simulink subsystem "kemba_simulation"  (R2022a)
settings: Solver=VariableStepAuto  StartTime=0.0  StopTime=10.0  RelTol=1e-3
values from neighbouring files (symbols this model uses):
  N = 6    [parameters.m]
undefined symbols (not defined in the file or in its folder): Body, Carrier, Femur, Piston, Ring, Tibia, X, Y, Z
libraries: sm_lib x95, nesl_utility x33, eeGeneralControl x4, Multibody_Parts_Lib x2, fl_lib x2
(part 4 of 4)

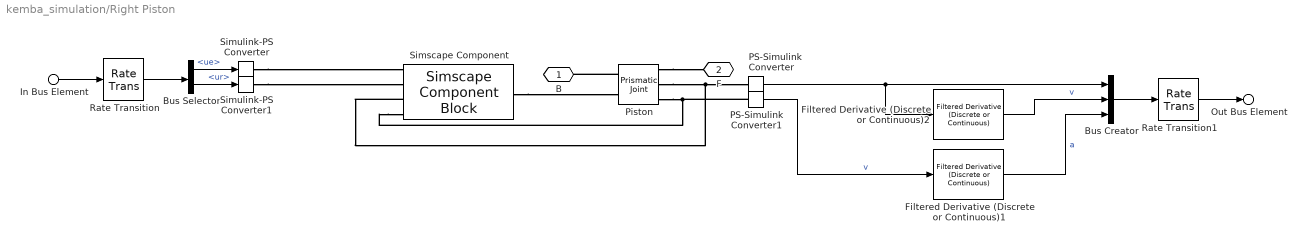
== system kemba_simulation/Right Piston ==
  In Bus Element : Inport  PortName=cmd
  Bus Creator : BusCreator  Inputs=3  OutDataTypeStr=Bus: PistonState
      settings: InheritFromInputs=off
  Bus Selector : BusSelector  OutputSignals=ue,ur
  Filtered Derivative (Discrete or Continuous)1 : eeGeneralControl/Filtered Derivative (Discrete or Continuous)  K=1  T=0.002  B=inf  A=-inf  minRatio=2  init_option=Inherited from block input  x0=0  Ts=-1
      settings: SourceProductBaseCode=PS
  Filtered Derivative (Discrete or Continuous)2 : eeGeneralControl/Filtered Derivative (Discrete or Continuous)  K=1  T=0.002  B=inf  A=-inf  minRatio=2  init_option=Inherited from block input  x0=0  Ts=-1
      settings: SourceProductBaseCode=PS
  PS-Simulink Converter : nesl_utility/PS-Simulink Converter  PhysicalDomain=network_engine_domain  SubClassName=ps_output  LeftPortType=input  RightPortType=output  PseudoPeriodic=off  Frequencies=[]  VectorFormat=inherit  Unit=inherit  AffineConversion=off
      settings: SourceProductBaseCode=SS,PW,VE
  PS-Simulink Converter1 : nesl_utility/PS-Simulink Converter  PhysicalDomain=network_engine_domain  SubClassName=ps_output  LeftPortType=input  RightPortType=output  PseudoPeriodic=off  Frequencies=[]  VectorFormat=inherit  Unit=inherit  AffineConversion=off
      settings: SourceProductBaseCode=SS,PW,VE
  Piston : sm_lib/Joints/Prismatic Joint  JointMode=Normal  SenseConstraintForce=off  SenseConstraintForceX=off  SenseConstraintForceY=off  SenseConstraintForceZ=off  SenseConstraintTorque=off  SenseConstraintTorqueX=off  SenseConstraintTorqueY=off  SenseConstraintTorqueZ=off  SenseTotalForce=off  SenseTotalForceX=off  SenseTotalForceY=off  SenseTotalForceZ=off  SenseTotalTorque=off  SenseTotalTorqueX=off  SenseTotalTorqueY=off  SenseTotalTorqueZ=off  CompositeWrenchDir=FollowerOnBase  CompositeWrenchFrame=BaseFrame  EquilibriumPosition=0  EquilibriumPositionUnits=m  SpringStiffness=0  SpringStiffnessUnits=N/m  DampingCoefficient=0  DampingCoefficientUnits=N/(m/s)  TorqueActuationMode=InputTorque  MotionActuationMode=ComputedMotion  SensePosition=on  SenseVelocity=on  SenseAcceleration=off  SenseTorqueForce=off  SenseLowerLimitTorqueForce=off  SenseUpperLimitTorqueForce=off  LowerLimitSpecify=on  LowerLimitBound=0  LowerLimitBoundUnits=m  LowerLimitStiffness=Piston.Limit.stiffness  LowerLimitStiffnessUnits=N/m  LowerLimitDamping=Piston.Limit.damping  LowerLimitDampingUnits=N/(m/s)  LowerLimitTransitionRegionWidth=Piston.Limit.transition_region_width  LowerLimitTransitionRegionWidthUnits=m  UpperLimitSpecify=on  UpperLimitBound=70  UpperLimitBoundUnits=mm  UpperLimitStiffness=Piston.Limit.stiffness  UpperLimitStiffnessUnits=N/m  UpperLimitDamping=Piston.Limit.damping  UpperLimitDampingUnits=N/(m/s)  UpperLimitTransitionRegionWidth=Piston.Limit.transition_region_width  UpperLimitTransitionRegionWidthUnits=m  PositionTargetSpecify=on  PositionTargetPriority=High  PositionTargetValue=Piston.Right.p0  PositionTargetValueUnits=m  VelocityTargetSpecify=on  VelocityTargetPriority=High  VelocityTargetValue=Piston.Right.v0  VelocityTargetValueUnits=m/s
  Rate Transition : RateTransition
  Rate Transition1 : RateTransition
  Simscape Component : SimscapeComponentBlock  SourceFile=PistonDynamics  ComponentPath=PistonDynamics  ComponentVariants="[\"PistonDynamics\"]"  ComponentVariantNames="[\"PistonDynamics\"]"  ClassName=PistonDynamics  SchemaVersion=1  Ps=7 bar  Pe=1 atm  Db=25 mm  Dr=10 mm  do=3 mm  td=6 ms  l=70 mm  kd=5 N  kv=25 N*s/m  T=295 K  R=286.71 J/(K*kg)  c=0.5  Z=0.99  k=1.4  v1=13069 mm^3  v2=16084 mm^3  P1_specify=off  P1_priority=None  P1=1 atm  P1_nominal_specify=off  P1_nominal_unit=atm  P1_nominal_value=1  P2_specify=off  P2_priority=None  P2=1 atm  P2_nominal_specify=off  P2_nominal_unit=atm  P2_nominal_value=1
      settings: CopyFcn=simscape.engine.sli.internal.componentblockcallback(gcbh,'COPY')  PreCopyFcn=simscape.engine.sli.internal.componentblockcallback(gcbh,'PRECOPY')  PreDeleteFcn=simscape.engine.sli.internal.componentblockcallback(gcbh,'PREDELETE')  LogSimulationData=on  InternalSimscapePortConfiguration="{\"Bottom\":[],\"Left\":[{\"id\":\"ue\",\"label\":\"ue\",\"type\":\"input\"},{\"id\":\"ur\",\"label\":\"ur\",\"type\":\"input\"},{\"id\":\"x\",\"label\":\"x\",\"type\":\"input\"},{\"id\":\"v\",\"label\":\"v\",\"type\":\"input\"}],\"Right\":[{\"id\":\"F\",\"label\":\"F\",\"type\":\"output\"}],\"Top\":[]}"
      mask Type: Piston Pressure Dynamics
  Simulink-PS Converter : nesl_utility/Simulink-PS Converter  PhysicalDomain=network_engine_domain  SubClassName=ps_input  LeftPortType=input  RightPortType=output  PseudoPeriodic=off  Frequencies=[]  NoiseDistribution=none  NoiseParameters=[]  Unit=1  AffineConversion=off  FilteringAndDerivatives=provide  SimscapeFilterOrder=1  InputFilterTimeConstant=0.001  UdotUserProvided=0
      settings: SourceProductBaseCode=SS,PW,VE
  Simulink-PS Converter1 : nesl_utility/Simulink-PS Converter  PhysicalDomain=network_engine_domain  SubClassName=ps_input  LeftPortType=input  RightPortType=output  PseudoPeriodic=off  Frequencies=[]  NoiseDistribution=none  NoiseParameters=[]  Unit=1  AffineConversion=off  FilteringAndDerivatives=provide  SimscapeFilterOrder=1  InputFilterTimeConstant=0.001  UdotUserProvided=0
      settings: SourceProductBaseCode=SS,PW,VE
  B : PMIOPort  Side=Left
  F : PMIOPort  Port=2  Side=Right
  Out Bus Element : Outport  PortName=state
  wires:
  Filtered Derivative (Discrete or Continuous)2/1 -> Bus Creator/2  "v"
  Filtered Derivative (Discrete or Continuous)1/1 -> Bus Creator/3  "a"
  Rate Transition1/1 -> Out Bus Element/1
  Bus Creator/1 -> Rate Transition1/1
  PS-Simulink Converter1/1 -> Filtered Derivative (Discrete or Continuous)1/1  "v"
  Bus Selector/1 -> Simulink-PS Converter/1  "<ue>"
  PS-Simulink Converter/1 -> Bus Creator/1, Filtered Derivative (Discrete or Continuous)2/1
  In Bus Element/1 -> Rate Transition/1
  Rate Transition/1 -> Bus Selector/1
  Bus Selector/2 -> Simulink-PS Converter1/1  "<ur>"
  connections:
  Simscape Component/LConn4 -- Piston/RConn3 -- PS-Simulink Converter1/LConn1
  Piston/RConn1 -- F/RConn1
  Piston/LConn1 -- B/RConn1
  Simscape Component/LConn3 -- Piston/RConn2 -- PS-Simulink Converter/LConn1
  Simulink-PS Converter/RConn1 -- Simscape Component/LConn1
  Simulink-PS Converter1/RConn1 -- Simscape Component/LConn2
  Simscape Component/RConn1 -- Piston/LConn2

== matlab function kemba_simulation/Left Motor/MATLAB Function ==
  data: cmd input; q input; t output; w input
function t = PD(cmd,q,w)
t = cmd.Kp*(cmd.q - q) + cmd.Kd*(cmd.w - w) + cmd.tff;

== matlab function kemba_simulation/Right Motor/MATLAB Function ==
  data: cmd input; q input; t output; w input
function t = PD(cmd,q,w)
t = cmd.Kp*(cmd.q - q) + cmd.Kd*(cmd.w - w) + cmd.tff;

== matlab function kemba_simulation/Planarising Boom/MATLAB Function ==
  data: roll_q input; roll_w input; pitch_q input; pitch_w input; pitch_b input; yaw_q input; state output Bus: BodyState; yaw_w input; yaw_b input
function state = boom_state(roll_q, roll_w, pitch_q, pitch_w, pitch_b, yaw_q, yaw_w, yaw_b)
pitchRadius = 2.493; % m
yawRadius = 2.575; % m
pitchHeightOffset = 0.101; % m

state.x = yawRadius * yaw_q;
state.dx = yawRadius * yaw_w;
state.ddx = yawRadius * yaw_b;

state.y = pitchRadius * sin(pitch_q) + pitchHeightOffset;
state.dy = pitchRadius * cos(pitch_q) * pitch_w;
state.ddy = pitchRadius * cos(pitch_q) * pitch_b - pitchRadius * sin(pitch_q) * pitch_w * pitch_w;

state.r = roll_q;
state.dr = roll_w;
end
